simulink model "untitled112"  (R2019a)
settings: Solver=VariableStepAuto  StartTime=0.0  StopTime=10.0  RelTol=1e-3
settings Model: Creator=wilso  LastModifiedBy=wilso

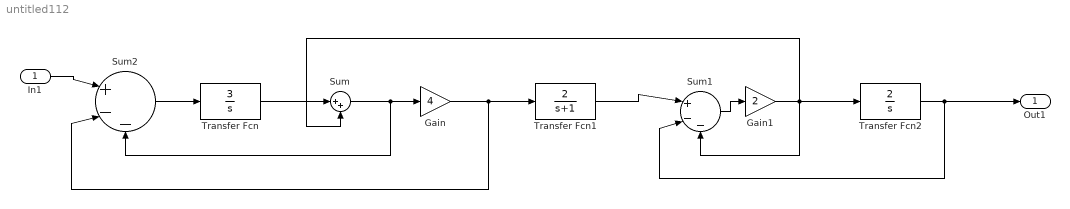
== system untitled112 ==
  In1 : Inport
  Gain : Gain  Gain=4
  Gain1 : Gain  Gain=2
  Sum : Sum  Inputs=|++
  Sum1 : Sum  Inputs=|+--
  Sum2 : Sum  Inputs=|+--
  Transfer Fcn : TransferFcn  Numerator=[3]  Denominator=[1 0]
  Transfer Fcn1 : TransferFcn  Numerator=[2]  Denominator=[1 1]
  Transfer Fcn2 : TransferFcn  Numerator=[2]  Denominator=[1 0]
  Out1 : Outport
  wires:
  Transfer Fcn/1 -> Sum/1
  Sum/1 -> Sum2/3, Gain/1
  Gain/1 -> Sum2/2, Transfer Fcn1/1
  Transfer Fcn1/1 -> Sum1/1
  Sum1/1 -> Gain1/1
  Sum2/1 -> Transfer Fcn/1
  Gain1/1 -> Sum1/3, Sum/2, Transfer Fcn2/1
  Transfer Fcn2/1 -> Out1/1, Sum1/2
  In1/1 -> Sum2/1
